simulink model "new_kalman"  (Simulink 7.1)
settings: Solver=ode4  StartTime=0.0  StopTime=1500  FixedStep=0.1  RelTol=1e-3
undefined symbols (not defined in the file or in its folder): kalmanfilter
libraries: fordypningsprosjekt x6, simulink x1
settings Model: Creator=anderga  LastModifiedBy=anderga

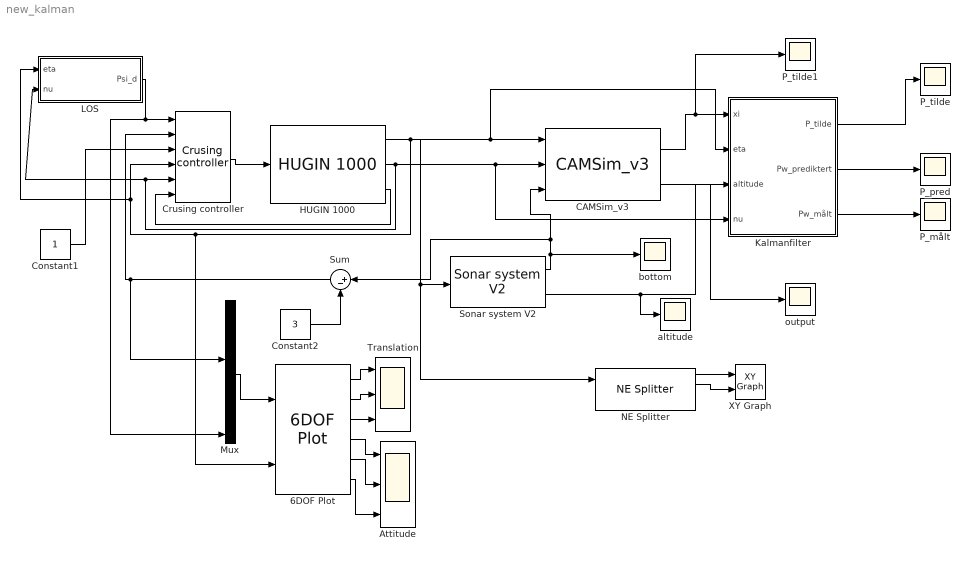
== system new_kalman ==
  6DOF Plot : fordypningsprosjekt/6DOF Plot  SystemSampleTime=-1
  Attitude : Scope  NumInputPorts=3
      settings: YMin=-0.3~-10~0  YMax=0.2~1~90  SaveName=Attitude
  CAMSim_v3 : fordypningsprosjekt/CAMSim_v3  SystemSampleTime=-1  noise=on  variance=0.01
  Constant1 : Constant  OutDataType=sfix(16)  OutScaling=2^0
  Constant2 : Constant  Value=3  OutDataType=sfix(16)  OutScaling=2^0
  Crusing controller : fordypningsprosjekt/Crusing controller  SystemSampleTime=-1  Kp_u=10  Ki_u=3  Kp_c=100  Kd_c=50  Kp_d=50  Kp2_d=20  Kd_d=20
  HUGIN 1000 : fordypningsprosjekt/HUGIN 1000  SystemSampleTime=-1  eta_0=[-30 0 0 0 0 0]  nu_0=[0 0 0 0 0 0]  c_on_off=off  beta_c=-45  V_c=0.3
  Kalmanfilter : Subsystem
  LOS : Subsystem  AncestorBlock=fordypningsprosjekt/LOS
  Mux : Mux  Inputs=6
  NE Splitter : fordypningsprosjekt/NE Splitter  SystemSampleTime=-1
  P_målt : Scope
      settings: YMin=-35  YMax=25  SaveName=Pipeline_malt
  P_pred : Scope
      settings: YMin=0  YMax=400  SaveName=Pipeline_pred
  P_tilde : Scope
      settings: YMin=-27.5  YMax=2.5
  P_tilde1 : Scope
      settings: YMin=-0.03  YMax=0.025  SaveName=Cam_output
  Sonar system V2 : fordypningsprosjekt/Sonar system V2  SystemSampleTime=-1  sea_bottom=-40
  Sum : Sum  Orientation=left  Inputs=|+-  OutDataType=sfix(16)  OutScaling=2^0
  Translation : Scope  NumInputPorts=3
      settings: YMin=-40~0~0  YMax=80~450~10  SaveName=Translation
  XY Graph : simulink/Sinks/XY Graph  SystemSampleTime=-1  xmin=-1000  xmax=1000  ymin=-1000  ymax=1000  st=-1
  altitude : Scope
      settings: YMin=3.4225  YMax=3.4525  SaveName=ScopeData6
  bottom : Scope
      settings: YMin=10.44  YMax=10.57  SaveName=ScopeData5
  output : Scope
      settings: YMin=0  YMax=1  SaveName=ScopeData3
  wires:
  HUGIN 1000/1 -> CAMSim_v3/1, Kalmanfilter/2(eta), 6DOF Plot/2, Crusing controller/4, LOS/1(eta), Sonar system V2/1, NE Splitter/1
  HUGIN 1000/2 -> CAMSim_v3/2, Kalmanfilter/4(nu), Crusing controller/5, LOS/2(nu)
  Sonar system V2/1 -> bottom/1, CAMSim_v3/3, Sum/1
  CAMSim_v3/1 -> Kalmanfilter/1(xi), P_tilde1/1
  Sonar system V2/2 -> Kalmanfilter/3(altitude), altitude/1
  Crusing controller/1 -> HUGIN 1000/1
  Kalmanfilter/1(P_tilde) -> P_tilde/1
  6DOF Plot/1 -> Translation/1
  6DOF Plot/2 -> Translation/2
  6DOF Plot/3 -> Translation/3
  6DOF Plot/4 -> Attitude/1
  6DOF Plot/5 -> Attitude/2
  6DOF Plot/6 -> Attitude/3
  HUGIN 1000/3 -> Crusing controller/6
  LOS/1(Psi_d) -> Crusing controller/1, Mux/6
  Constant1/1 -> Crusing controller/3
  Mux/1 -> 6DOF Plot/1
  NE Splitter/1 -> XY Graph/1
  NE Splitter/2 -> XY Graph/2
  Kalmanfilter/2(Pw_prediktert) -> P_pred/1
  Kalmanfilter/3(Pw_målt) -> P_målt/1
  CAMSim_v3/2 -> output/1
  Constant2/1 -> Sum/2
  Sum/1 -> Crusing controller/2, Mux/3

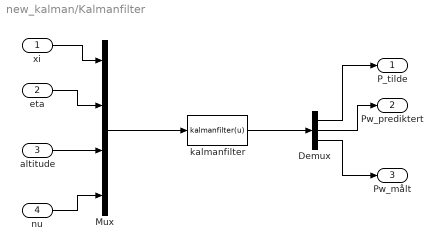
== system new_kalman/Kalmanfilter ==
  xi : Inport  OutDataType=sfix(16)  OutScaling=2^0
  eta : Inport  Port=2  OutDataType=sfix(16)  OutScaling=2^0
  altitude : Inport  Port=3  OutDataType=sfix(16)  OutScaling=2^0
  nu : Inport  Port=4  OutDataType=sfix(16)  OutScaling=2^0
  Demux : Demux  Outputs=3
  Mux : Mux
  kalmanfilter : MATLABFcn  MATLABFcn=kalmanfilter(u)  OutputDimensions=9
  P_tilde : Outport  OutDataType=sfix(16)  OutScaling=2^0
  Pw_prediktert : Outport  Port=2  OutDataType=sfix(16)  OutScaling=2^0
  Pw_målt : Outport  Port=3  OutDataType=sfix(16)  OutScaling=2^0
  wires:
  xi/1 -> Mux/1
  eta/1 -> Mux/2
  altitude/1 -> Mux/3
  nu/1 -> Mux/4
  Mux/1 -> kalmanfilter/1
  kalmanfilter/1 -> Demux/1
  Demux/1 -> P_tilde/1
  Demux/2 -> Pw_prediktert/1
  Demux/3 -> Pw_målt/1

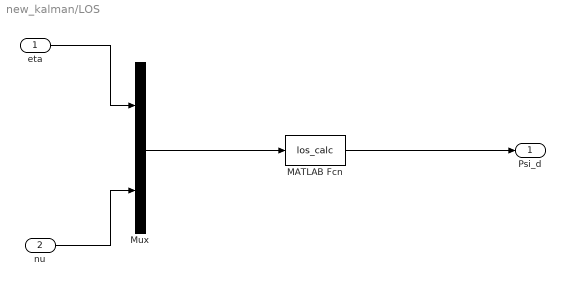
== system new_kalman/LOS ==
  eta : Inport  OutDataType=sfix(16)  OutScaling=2^0
  nu : Inport  Port=2  OutDataType=sfix(16)  OutScaling=2^0
  MATLAB Fcn : MATLABFcn  MATLABFcn=los_calc  OutputDimensions=1
  Mux : Mux  Inputs=2
  Psi_d : Outport  OutDataType=sfix(16)  OutScaling=2^0
  wires:
  eta/1 -> Mux/1
  nu/1 -> Mux/2
  Mux/1 -> MATLAB Fcn/1
  MATLAB Fcn/1 -> Psi_d/1
